simulink model "randomControllerSim3"  (R2015b)
settings: Solver=VariableStepAuto  StartTime=0.0  StopTime=1.5  FixedStep=1/10000  RelTol=1e-6
values from neighbouring files (symbols this model uses):
  B_f = 7.7e-3    (= 0.0077)    [randomController.m]
  B_w = 17.03e-6    (= 1.703e-05)    [randomController.m]
  disturb = 0.55    [randomController.m]
  g = 9.82    [randomController.m]
  J_f = 4.8e-3    (= 0.0048)    [randomController.m]
  J_w = 0.601e-3    (= 0.000601)    [randomController.m]
  l_f = 0.08498    [randomController.m]
  l_w = 0.093    [randomController.m]
  m_f = 0.77-m_w    (= 0.548)    [randomController.m]
  m_w = 0.222    [randomController.m]
  t_dist = 0.01    [randomController.m]
settings Model: Creator=USUARIO  LastModifiedBy=USUARIO
settings DataIOCC: LimitDataPoints=off  SaveFormat=Array  SignalLoggingSaveFormat=ModelDataLogs
settings DebuggingCC: SolverPrmCheckMsg=warning
settings HardwareCC: ProdBitPerPointer=32  ProdLargestAtomicFloat=None  ProdIntDivRoundTo=Undefined  ProdEndianess=Unspecified  ProdWordSize=32  ProdHWDeviceType=32-bit Generic
settings GRTTargetCC: GeneratePreprocessorConditionals=Disable all
settings ConfigComp: CovModelRefEnable=Off  CovSFcnEnable=off

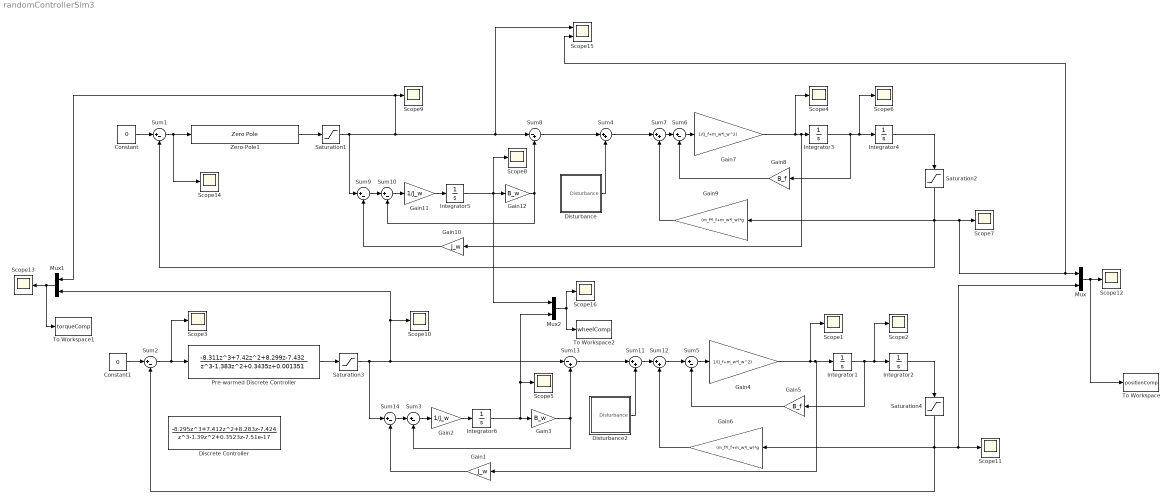
== system randomControllerSim3 ==
  Constant : Constant  Value=0
  Constant1 : Constant  Value=0
  Discrete Controller : DiscreteTransferFcn  Numerator=[-8.295 7.412 8.283 -7.424]  Denominator=[1 -1.39 0.3523 -7.51e-17]  SampleTime=1/100
  Disturbance : Subsystem
  Disturbance2 : Subsystem
  Gain1 : Gain  Gain=J_w
  Gain10 : Gain  Gain=J_w
  Gain11 : Gain  Gain=1/J_w
  Gain12 : Gain  Gain=B_w
  Gain2 : Gain  Gain=1/J_w
  Gain3 : Gain  Gain=B_w
  Gain4 : Gain  Gain=1/(J_f+m_w*l_w^2)
  Gain5 : Gain  Gain=B_f
  Gain6 : Gain  Gain=(m_f*l_f+m_w*l_w)*g
  Gain7 : Gain  Gain=1/(J_f+m_w*l_w^2)
  Gain8 : Gain  Gain=B_f
  Gain9 : Gain  Gain=(m_f*l_f+m_w*l_w)*g
  Integrator{1..6} (6 alike) : Integrator
  Mux : Mux  Inputs=2
  Mux1 : Mux  Inputs=2
  Mux2 : Mux  Inputs=2
  Pre-warmed Discrete Controller : DiscreteTransferFcn  Numerator=[-8.311 7.42 8.299 -7.432]  Denominator=[1 -1.383 0.3435 0.001351]  SampleTime=1/100
  Saturation1 : Saturate  UpperLimit=4*0.0335  LowerLimit=-4*0.0335
  Saturation2 : Saturate  UpperLimit=0.85  LowerLimit=-0.72
  Saturation3 : Saturate  UpperLimit=4*0.0335  LowerLimit=-4*0.0335
  Saturation4 : Saturate  UpperLimit=0.85  LowerLimit=-0.72
  Scope{1..14,16} (15 alike) : Scope
  Scope15 : Scope  NumInputPorts=2
  Sum{1..3,5..6,9..10,14} (8 alike) : Sum  Inputs=|+-
  Sum{4,7,11..12} (4 alike) : Sum  Inputs=|++
  Sum13 : Sum  Inputs=|-+
  Sum8 : Sum  Inputs=|-+
  To Workspace : ToWorkspace  VariableName=positionComp  SaveFormat=Timeseries  SampleTime=-1
  To Workspace1 : ToWorkspace  VariableName=torqueComp  SaveFormat=Timeseries  SampleTime=-1
  To Workspace2 : ToWorkspace  VariableName=wheelComp  SaveFormat=Timeseries  SampleTime=-1
  Zero-Pole1 : ZeroPole  Zeros=[-9.483 -1.599]  Poles=[-200 -100 5.539]  Gain=[-0.62737*200*100*5.539/9.483/1.599]
  wires:
  Gain7/1 -> Scope4/1, Gain10/1, Integrator3/1
  Integrator3/1 -> Gain8/1, Scope6/1, Integrator4/1
  Sum6/1 -> Gain7/1
  Sum7/1 -> Sum6/1
  Gain8/1 -> Sum6/2
  Gain9/1 -> Sum7/2
  Sum10/1 -> Gain11/1
  Gain11/1 -> Integrator5/1
  Gain10/1 -> Sum9/2
  Sum9/1 -> Sum10/1
  Integrator5/1 -> Mux2/1, Scope8/1, Gain12/1
  Gain12/1 -> Sum10/2, Sum8/2
  Integrator4/1 -> Saturation2/1
  Sum1/1 -> Scope14/1, Zero-Pole1/1
  Saturation1/1 -> Scope15/1, Sum8/1, Mux1/1, Scope9/1, Sum9/1
  Gain4/1 -> Gain1/1, Integrator1/1, Scope1/1
  Integrator1/1 -> Gain5/1, Scope2/1, Integrator2/1
  Sum5/1 -> Gain4/1
  Sum12/1 -> Sum5/1
  Gain5/1 -> Sum5/2
  Gain6/1 -> Sum12/2
  Sum3/1 -> Gain2/1
  Gain2/1 -> Integrator6/1
  Gain1/1 -> Sum14/2
  Sum14/1 -> Sum3/1
  Integrator6/1 -> Mux2/2, Scope5/1, Gain3/1
  Gain3/1 -> Sum3/2, Sum13/2
  Sum2/1 -> Scope3/1, Pre-warmed Discrete Controller/1
  Mux/1 -> To Workspace/1, Scope12/1
  Saturation3/1 -> Sum13/1, Scope10/1, Mux1/2, Sum14/1
  Mux1/1 -> To Workspace1/1, Scope13/1
  Integrator2/1 -> Saturation4/1
  Saturation4/1 -> Sum2/2, Gain6/1, Mux/2, Scope11/1
  Saturation2/1 -> Gain9/1, Scope7/1, Mux/1, Scope15/2, Sum1/2
  Constant/1 -> Sum1/1
  Constant1/1 -> Sum2/1
  Zero-Pole1/1 -> Saturation1/1
  Pre-warmed Discrete Controller/1 -> Saturation3/1
  Mux2/1 -> Scope16/1, To Workspace2/1
  Disturbance/1(Disturbance) -> Sum4/2
  Sum4/1 -> Sum7/1
  Sum8/1 -> Sum4/1
  Disturbance2/1(Disturbance) -> Sum11/2
  Sum11/1 -> Sum12/1
  Sum13/1 -> Sum11/1

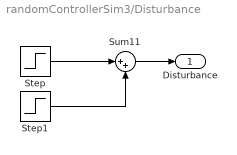
== system randomControllerSim3/Disturbance ==
  Step : Step  Time=0.1  After=disturb  SampleTime=0
  Step1 : Step  Time=0.1+t_dist  After=-disturb  SampleTime=0
  Sum11 : Sum  Inputs=|++
  Disturbance : Outport
  wires:
  Step1/1 -> Sum11/2
  Step/1 -> Sum11/1
  Sum11/1 -> Disturbance/1

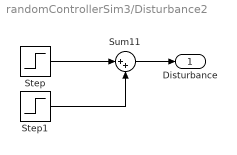
== system randomControllerSim3/Disturbance2 ==
  Step : Step  Time=0.1  After=disturb  SampleTime=0
  Step1 : Step  Time=0.1+t_dist  After=-disturb  SampleTime=0
  Sum11 : Sum  Inputs=|++
  Disturbance : Outport
  wires:
  Sum11/1 -> Disturbance/1
  Step/1 -> Sum11/1
  Step1/1 -> Sum11/2
